simulink model "a"  (R2016a)
settings: Solver=VariableStepAuto  StartTime=0.0  StopTime=10.0  RelTol=1e-3
settings Model: Creator=hp  LastModifiedBy=hp

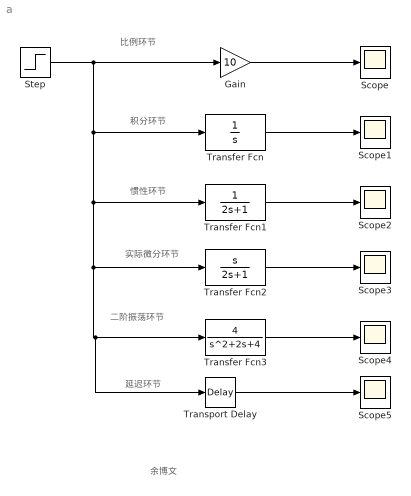
== system a ==
  note: 余博文
  note: 延迟环节
  note: 惯性环节
  note: 积分环节
  note: 比例环节
  note: 实际微分环节
  note: 二阶振荡环节
  Gain : Gain  Gain=10
  Scope{,1..5} (6 alike) : Scope
  Step : Step  SampleTime=0
  Transfer Fcn : TransferFcn  Denominator=[1 0]
  Transfer Fcn1 : TransferFcn  Denominator=[2 1]
  Transfer Fcn2 : TransferFcn  Numerator=[1 0]  Denominator=[2 1]
  Transfer Fcn3 : TransferFcn  Numerator=[4]  Denominator=[1 2 4]
  Transport Delay : TransportDelay  DelayTime=2
  wires:
  Gain/1 -> Scope/1
  Transfer Fcn/1 -> Scope1/1
  Transfer Fcn1/1 -> Scope2/1
  Transfer Fcn2/1 -> Scope3/1
  Step/1 -> Transport Delay/1, Transfer Fcn3/1, Transfer Fcn2/1, Transfer Fcn1/1, Transfer Fcn/1, Gain/1
  Transfer Fcn3/1 -> Scope4/1
  Transport Delay/1 -> Scope5/1
